simulink model "ElectricCircuit"  (R2019b)
settings: Solver=ode45  StartTime=0.0  StopTime=20.0  MaxStep=0.01  MinStep=0.001  RelTol=1e-3
settings Model: Creator=Lenovo  LastModifiedBy=Lenovo

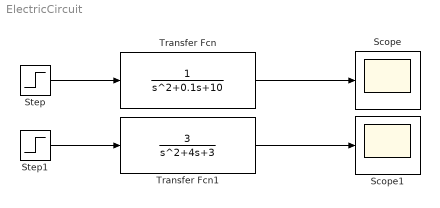
== system ElectricCircuit ==
  Scope : Scope
  Scope1 : Scope
  Step : Step  SampleTime=0
  Step1 : Step  SampleTime=0
  Transfer Fcn : TransferFcn  Denominator=[1 0.1 10]
  Transfer Fcn1 : TransferFcn  Numerator=[3]  Denominator=[1 4 3]
  wires:
  Transfer Fcn/1 -> Scope/1
  Step/1 -> Transfer Fcn/1
  Step1/1 -> Transfer Fcn1/1
  Transfer Fcn1/1 -> Scope1/1
